simulink model "project_part4_simulink"  (R2025b)
settings: Solver=VariableStepAuto  StartTime=0.0  StopTime=60000  RelTol=1e-3
values from neighbouring files (symbols this model uses):
  denLL = [1 1.14727809e-02 9.96311098e-07]    [Projectpart4_matlab.m]
  Kd = 7.622663874609e-03    (= 0.00762266387461)    [Projectpart4_matlab.m]
  Ki = 2.615765353720e-08    (= 2.61576535372e-08)    [Projectpart4_matlab.m]
  Kp = 5.084451890329e-05    (= 5.08445189033e-05)    [Projectpart4_matlab.m]
  N = 4.500000000000e-02    (= 0.045)    [Projectpart4_matlab.m]
  numLL = [1.73797606e-04 5.57358725e-07 2.53973523e-10]    [Projectpart4_matlab.m]
  Td = 11.7    [Projectpart4_matlab.m]
libraries: slpidlib x10, simulink x2
settings Model: PacingRate=1000  Creator=DELL  LastModifiedBy=renef

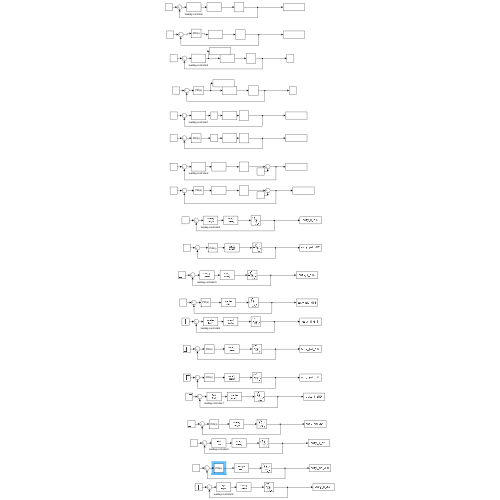
[thumbnail: Simulink's stored preview of the top-level diagram]
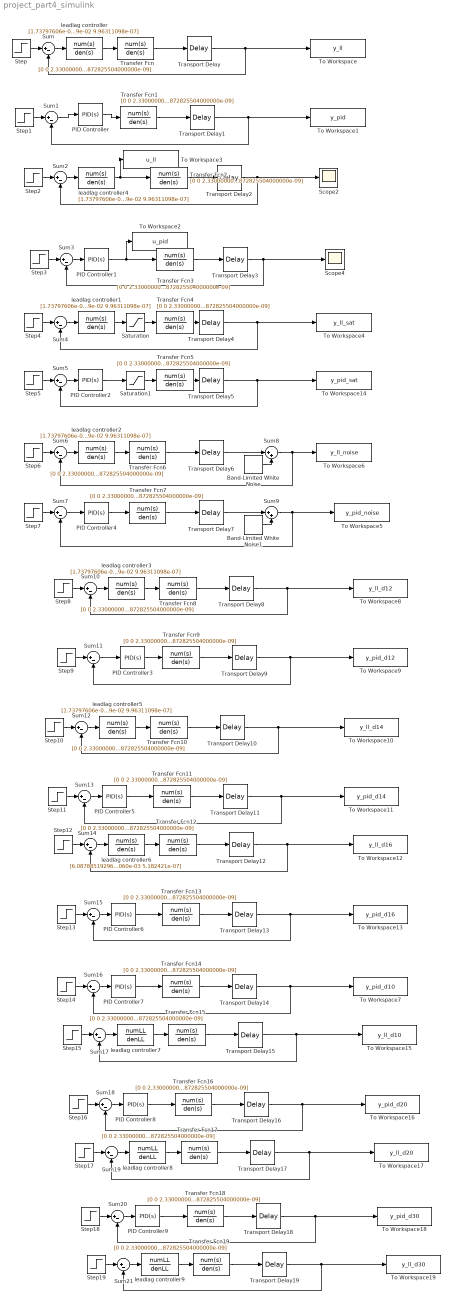
== system project_part4_simulink ==
  Band-Limited White Noise : simulink/Sources/Band-Limited White Noise  Cov=[0.001]  Ts=1  seed=[23341]
  Band-Limited White Noise1 : simulink/Sources/Band-Limited White Noise  Cov=[0.001]  Ts=1  seed=[23341]
  PID Controller{,1..6} (7 alike) : slpidlib/PID Controller  Controller=PID  Form=Parallel  TimeDomain=Continuous-time  UseExternalTs=off  SampleTime=-1  IntegratorMethod=Forward Euler  FilterMethod=Forward Euler  ControllerParametersSource=internal  P=5.084451890329e-05  I=2.615765353720e-08  UseKiTs=off  D=7.622663874609e-03  UseExternalDerivativeSource=off  N=4.500000000000e-02  UseFilter=on  TunerSelectOption=Transfer Function Based (PID Tuner App)  InitialConditionSource=internal  InitialConditionForIntegrator=0  InitialConditionForFilter=0  DifferentiatorICPrevScaledInput=0  ExternalReset=none  TrackingMode=off  Kt=1  LimitOutput=off  SatLimitsSource=internal  UpperSaturationLimit=inf  LowerSaturationLimit=-inf  LinearizeAsGain=on  AntiWindupMode=none  Kb=1  LimitIntegrator=off  UpperIntegratorSaturationLimit=inf  LowerIntegratorSaturationLimit=-inf  POutMin=[]  POutMax=[]  IOutMin=[]  IOutMax=[]  DOutMin=[]  DOutMax=[]  NOutMin=[]  NOutMax=[]  SumOutMin=[]  SumOutMax=[]  SaturationOutMin=[]  SaturationOutMax=[]  PParamMin=[]  PParamMax=[]  IParamMin=[]  IParamMax=[]  DParamMin=[]  DParamMax=[]  NParamMin=[]  NParamMax=[]  KbParamMin=[]  KbParamMax=[]  KtParamMin=[]  KtParamMax=[]  KbOutMin=[]  KbOutMax=[]  KtOutMin=[]  KtOutMax=[]  IntegratorOutMin=[]  IntegratorOutMax=[]  FilterOutMin=[]  FilterOutMax=[]  SumI1OutMin=[]  SumI1OutMax=[]  SumI2OutMin=[]  SumI2OutMax=[]  SumI3OutMin=[]  SumI3OutMax=[]  SumI4OutMin=[]  SumI4OutMax=[]  SumDOutMin=[]  SumDOutMax=[]  DifferentiatorOutMin=[]  DifferentiatorOutMax=[]  FilterDiffOutCoefMin=[]  FilterDiffOutCoefMax=[]  ReciprocalOutMin=[]  ReciprocalOutMax=[]  SumDenOutMin=[]  SumDenOutMax=[]  SumNumOutMin=[]  SumNumOutMax=[]  DivideOutMin=[]  DivideOutMax=[]  UdiffTsProdOutMin=[]  UdiffTsProdOutMax=[]  NTsProdOutMin=[]  NTsProdOutMax=[]  UintegralTsProdOutMin=[]  UintegralTsProdOutMax=[]  UngainTsProdOutMin=[]  UngainTsProdOutMax=[]  ClampingZeroOutDataTypeStr=Inherit: Inherit via back propagation  ClampingZeroOutMin=[]  ClampingZeroOutMax=[]  FilterDenConstantOutDataTypeStr=Inherit: Inherit via back propagation  FilterDenConstantOutMin=[]  FilterDenConstantOutMax=[]  PCopyOutDataTypeStr=Inherit: Inherit via back propagation  PCopyOutMin=[]  PCopyOutMax=[]  NCopyOutDataTypeStr=Inherit: Inherit via back propagation  NCopyOutMin=[]  NCopyOutMax=[]  IntegratorContinuousStateAttributes=''  IntegratorStateMustResolveToSignalObject=off  IntegratorRTWStateStorageClass=Auto  FilterContinuousStateAttributes=''  FilterStateMustResolveToSignalObject=off  FilterRTWStateStorageClass=Auto  ParallelPVariant=InternalParameters  IdealPVariant=Disabled  IVariant=InternalParameters  DVariant=InternalParameters  IntegratorVariant=Continuous  SatVariant=Disabled  AWVariant=Passthrough  PCopyVariant=Disabled  TRVariant=Disabled  FdbkBlocksVariant=Forward  IdealPFdbkVariant=Disabled  SatFdbkVariant=Disabled  DerivativeFilterVariant=ContFilter  NVariant=InternalParameters  NCopyVariant=Disabled  FilterICVariant=InternalICsFilter  IntegratorICVariant=InternalICs  ExternalResetVariant=Disabled  TRSumVariant=Passthrough  SumFdbkVariant=Disabled  SumVariant=Sum_PID  TsampFilterVariant=InternalTs  TsampNgainVariant=Passthrough  TsampIntegralVariant=Disabled_SignalSpec  ExternalSaturationOutDataTypeStr=Inherit: Same as second input  DerivativeSourceVariant=ErrorSignal  PreIntVariant=InternalPreInt
  PID Controller7 : slpidlib/PID Controller  Controller=PID  Form=Parallel  TimeDomain=Continuous-time  UseExternalTs=off  SampleTime=-1  IntegratorMethod=Forward Euler  FilterMethod=Forward Euler  ControllerParametersSource=internal  P=Kp  I=Ki  UseKiTs=off  D=Kd  UseExternalDerivativeSource=off  N=N  UseFilter=on  TunerSelectOption=Transfer Function Based (PID Tuner App)  InitialConditionSource=internal  InitialConditionForIntegrator=0  InitialConditionForFilter=0  DifferentiatorICPrevScaledInput=0  ExternalReset=none  TrackingMode=off  Kt=1  LimitOutput=off  SatLimitsSource=internal  UpperSaturationLimit=inf  LowerSaturationLimit=-inf  LinearizeAsGain=on  AntiWindupMode=none  Kb=1  LimitIntegrator=off  UpperIntegratorSaturationLimit=inf  LowerIntegratorSaturationLimit=-inf  POutMin=[]  POutMax=[]  IOutMin=[]  IOutMax=[]  DOutMin=[]  DOutMax=[]  NOutMin=[]  NOutMax=[]  SumOutMin=[]  SumOutMax=[]  SaturationOutMin=[]  SaturationOutMax=[]  PParamMin=[]  PParamMax=[]  IParamMin=[]  IParamMax=[]  DParamMin=[]  DParamMax=[]  NParamMin=[]  NParamMax=[]  KbParamMin=[]  KbParamMax=[]  KtParamMin=[]  KtParamMax=[]  KbOutMin=[]  KbOutMax=[]  KtOutMin=[]  KtOutMax=[]  IntegratorOutMin=[]  IntegratorOutMax=[]  FilterOutMin=[]  FilterOutMax=[]  SumI1OutMin=[]  SumI1OutMax=[]  SumI2OutMin=[]  SumI2OutMax=[]  SumI3OutMin=[]  SumI3OutMax=[]  SumI4OutMin=[]  SumI4OutMax=[]  SumDOutMin=[]  SumDOutMax=[]  DifferentiatorOutMin=[]  DifferentiatorOutMax=[]  FilterDiffOutCoefMin=[]  FilterDiffOutCoefMax=[]  ReciprocalOutMin=[]  ReciprocalOutMax=[]  SumDenOutMin=[]  SumDenOutMax=[]  SumNumOutMin=[]  SumNumOutMax=[]  DivideOutMin=[]  DivideOutMax=[]  UdiffTsProdOutMin=[]  UdiffTsProdOutMax=[]  NTsProdOutMin=[]  NTsProdOutMax=[]  UintegralTsProdOutMin=[]  UintegralTsProdOutMax=[]  UngainTsProdOutMin=[]  UngainTsProdOutMax=[]  ClampingZeroOutDataTypeStr=Inherit: Inherit via back propagation  ClampingZeroOutMin=[]  ClampingZeroOutMax=[]  FilterDenConstantOutDataTypeStr=Inherit: Inherit via back propagation  FilterDenConstantOutMin=[]  FilterDenConstantOutMax=[]  PCopyOutDataTypeStr=Inherit: Inherit via back propagation  PCopyOutMin=[]  PCopyOutMax=[]  NCopyOutDataTypeStr=Inherit: Inherit via back propagation  NCopyOutMin=[]  NCopyOutMax=[]  IntegratorContinuousStateAttributes=''  IntegratorStateMustResolveToSignalObject=off  IntegratorRTWStateStorageClass=Auto  FilterContinuousStateAttributes=''  FilterStateMustResolveToSignalObject=off  FilterRTWStateStorageClass=Auto  ParallelPVariant=InternalParameters  IdealPVariant=Disabled  IVariant=InternalParameters  DVariant=InternalParameters  IntegratorVariant=Continuous  SatVariant=Disabled  AWVariant=Passthrough  PCopyVariant=Disabled  TRVariant=Disabled  FdbkBlocksVariant=Forward  IdealPFdbkVariant=Disabled  SatFdbkVariant=Disabled  DerivativeFilterVariant=ContFilter  NVariant=InternalParameters  NCopyVariant=Disabled  FilterICVariant=InternalICsFilter  IntegratorICVariant=InternalICs  ExternalResetVariant=Disabled  TRSumVariant=Passthrough  SumFdbkVariant=Disabled  SumVariant=Sum_PID  TsampFilterVariant=InternalTs  TsampNgainVariant=Passthrough  TsampIntegralVariant=Disabled_SignalSpec  ExternalSaturationOutDataTypeStr=Inherit: Same as second input  DerivativeSourceVariant=ErrorSignal  PreIntVariant=InternalPreInt
  PID Controller8 : slpidlib/PID Controller  Controller=PID  Form=Parallel  TimeDomain=Continuous-time  UseExternalTs=off  SampleTime=-1  IntegratorMethod=Forward Euler  FilterMethod=Forward Euler  ControllerParametersSource=internal  P=Kp  I=Ki  UseKiTs=off  D=Kd  UseExternalDerivativeSource=off  N=N  UseFilter=on  TunerSelectOption=Transfer Function Based (PID Tuner App)  InitialConditionSource=internal  InitialConditionForIntegrator=0  InitialConditionForFilter=0  DifferentiatorICPrevScaledInput=0  ExternalReset=none  TrackingMode=off  Kt=1  LimitOutput=off  SatLimitsSource=internal  UpperSaturationLimit=inf  LowerSaturationLimit=-inf  LinearizeAsGain=on  AntiWindupMode=none  Kb=1  LimitIntegrator=off  UpperIntegratorSaturationLimit=inf  LowerIntegratorSaturationLimit=-inf  POutMin=[]  POutMax=[]  IOutMin=[]  IOutMax=[]  DOutMin=[]  DOutMax=[]  NOutMin=[]  NOutMax=[]  SumOutMin=[]  SumOutMax=[]  SaturationOutMin=[]  SaturationOutMax=[]  PParamMin=[]  PParamMax=[]  IParamMin=[]  IParamMax=[]  DParamMin=[]  DParamMax=[]  NParamMin=[]  NParamMax=[]  KbParamMin=[]  KbParamMax=[]  KtParamMin=[]  KtParamMax=[]  KbOutMin=[]  KbOutMax=[]  KtOutMin=[]  KtOutMax=[]  IntegratorOutMin=[]  IntegratorOutMax=[]  FilterOutMin=[]  FilterOutMax=[]  SumI1OutMin=[]  SumI1OutMax=[]  SumI2OutMin=[]  SumI2OutMax=[]  SumI3OutMin=[]  SumI3OutMax=[]  SumI4OutMin=[]  SumI4OutMax=[]  SumDOutMin=[]  SumDOutMax=[]  DifferentiatorOutMin=[]  DifferentiatorOutMax=[]  FilterDiffOutCoefMin=[]  FilterDiffOutCoefMax=[]  ReciprocalOutMin=[]  ReciprocalOutMax=[]  SumDenOutMin=[]  SumDenOutMax=[]  SumNumOutMin=[]  SumNumOutMax=[]  DivideOutMin=[]  DivideOutMax=[]  UdiffTsProdOutMin=[]  UdiffTsProdOutMax=[]  NTsProdOutMin=[]  NTsProdOutMax=[]  UintegralTsProdOutMin=[]  UintegralTsProdOutMax=[]  UngainTsProdOutMin=[]  UngainTsProdOutMax=[]  ClampingZeroOutDataTypeStr=Inherit: Inherit via back propagation  ClampingZeroOutMin=[]  ClampingZeroOutMax=[]  FilterDenConstantOutDataTypeStr=Inherit: Inherit via back propagation  FilterDenConstantOutMin=[]  FilterDenConstantOutMax=[]  PCopyOutDataTypeStr=Inherit: Inherit via back propagation  PCopyOutMin=[]  PCopyOutMax=[]  NCopyOutDataTypeStr=Inherit: Inherit via back propagation  NCopyOutMin=[]  NCopyOutMax=[]  IntegratorContinuousStateAttributes=''  IntegratorStateMustResolveToSignalObject=off  IntegratorRTWStateStorageClass=Auto  FilterContinuousStateAttributes=''  FilterStateMustResolveToSignalObject=off  FilterRTWStateStorageClass=Auto  ParallelPVariant=InternalParameters  IdealPVariant=Disabled  IVariant=InternalParameters  DVariant=InternalParameters  IntegratorVariant=Continuous  SatVariant=Disabled  AWVariant=Passthrough  PCopyVariant=Disabled  TRVariant=Disabled  FdbkBlocksVariant=Forward  IdealPFdbkVariant=Disabled  SatFdbkVariant=Disabled  DerivativeFilterVariant=ContFilter  NVariant=InternalParameters  NCopyVariant=Disabled  FilterICVariant=InternalICsFilter  IntegratorICVariant=InternalICs  ExternalResetVariant=Disabled  TRSumVariant=Passthrough  SumFdbkVariant=Disabled  SumVariant=Sum_PID  TsampFilterVariant=InternalTs  TsampNgainVariant=Passthrough  TsampIntegralVariant=Disabled_SignalSpec  ExternalSaturationOutDataTypeStr=Inherit: Same as second input  DerivativeSourceVariant=ErrorSignal  PreIntVariant=InternalPreInt
  PID Controller9 : slpidlib/PID Controller  Controller=PID  Form=Parallel  TimeDomain=Continuous-time  UseExternalTs=off  SampleTime=-1  IntegratorMethod=Forward Euler  FilterMethod=Forward Euler  ControllerParametersSource=internal  P=Kp  I=Ki  UseKiTs=off  D=Kd  UseExternalDerivativeSource=off  N=N  UseFilter=on  TunerSelectOption=Transfer Function Based (PID Tuner App)  InitialConditionSource=internal  InitialConditionForIntegrator=0  InitialConditionForFilter=0  DifferentiatorICPrevScaledInput=0  ExternalReset=none  TrackingMode=off  Kt=1  LimitOutput=off  SatLimitsSource=internal  UpperSaturationLimit=inf  LowerSaturationLimit=-inf  LinearizeAsGain=on  AntiWindupMode=none  Kb=1  LimitIntegrator=off  UpperIntegratorSaturationLimit=inf  LowerIntegratorSaturationLimit=-inf  POutMin=[]  POutMax=[]  IOutMin=[]  IOutMax=[]  DOutMin=[]  DOutMax=[]  NOutMin=[]  NOutMax=[]  SumOutMin=[]  SumOutMax=[]  SaturationOutMin=[]  SaturationOutMax=[]  PParamMin=[]  PParamMax=[]  IParamMin=[]  IParamMax=[]  DParamMin=[]  DParamMax=[]  NParamMin=[]  NParamMax=[]  KbParamMin=[]  KbParamMax=[]  KtParamMin=[]  KtParamMax=[]  KbOutMin=[]  KbOutMax=[]  KtOutMin=[]  KtOutMax=[]  IntegratorOutMin=[]  IntegratorOutMax=[]  FilterOutMin=[]  FilterOutMax=[]  SumI1OutMin=[]  SumI1OutMax=[]  SumI2OutMin=[]  SumI2OutMax=[]  SumI3OutMin=[]  SumI3OutMax=[]  SumI4OutMin=[]  SumI4OutMax=[]  SumDOutMin=[]  SumDOutMax=[]  DifferentiatorOutMin=[]  DifferentiatorOutMax=[]  FilterDiffOutCoefMin=[]  FilterDiffOutCoefMax=[]  ReciprocalOutMin=[]  ReciprocalOutMax=[]  SumDenOutMin=[]  SumDenOutMax=[]  SumNumOutMin=[]  SumNumOutMax=[]  DivideOutMin=[]  DivideOutMax=[]  UdiffTsProdOutMin=[]  UdiffTsProdOutMax=[]  NTsProdOutMin=[]  NTsProdOutMax=[]  UintegralTsProdOutMin=[]  UintegralTsProdOutMax=[]  UngainTsProdOutMin=[]  UngainTsProdOutMax=[]  ClampingZeroOutDataTypeStr=Inherit: Inherit via back propagation  ClampingZeroOutMin=[]  ClampingZeroOutMax=[]  FilterDenConstantOutDataTypeStr=Inherit: Inherit via back propagation  FilterDenConstantOutMin=[]  FilterDenConstantOutMax=[]  PCopyOutDataTypeStr=Inherit: Inherit via back propagation  PCopyOutMin=[]  PCopyOutMax=[]  NCopyOutDataTypeStr=Inherit: Inherit via back propagation  NCopyOutMin=[]  NCopyOutMax=[]  IntegratorContinuousStateAttributes=''  IntegratorStateMustResolveToSignalObject=off  IntegratorRTWStateStorageClass=Auto  FilterContinuousStateAttributes=''  FilterStateMustResolveToSignalObject=off  FilterRTWStateStorageClass=Auto  ParallelPVariant=InternalParameters  IdealPVariant=Disabled  IVariant=InternalParameters  DVariant=InternalParameters  IntegratorVariant=Continuous  SatVariant=Disabled  AWVariant=Passthrough  PCopyVariant=Disabled  TRVariant=Disabled  FdbkBlocksVariant=Forward  IdealPFdbkVariant=Disabled  SatFdbkVariant=Disabled  DerivativeFilterVariant=ContFilter  NVariant=InternalParameters  NCopyVariant=Disabled  FilterICVariant=InternalICsFilter  IntegratorICVariant=InternalICs  ExternalResetVariant=Disabled  TRSumVariant=Passthrough  SumFdbkVariant=Disabled  SumVariant=Sum_PID  TsampFilterVariant=InternalTs  TsampNgainVariant=Passthrough  TsampIntegralVariant=Disabled_SignalSpec  ExternalSaturationOutDataTypeStr=Inherit: Same as second input  DerivativeSourceVariant=ErrorSignal  PreIntVariant=InternalPreInt
  Saturation : Saturate  UpperLimit=2e-5  LowerLimit=0
  Saturation1 : Saturate  UpperLimit=2e-5  LowerLimit=0
  Scope2 : Scope
      settings: ActiveDisplayYMinimum=-1  ActiveDisplayYMaximum=1  DataLoggingVariableName=ScopeData2
  Scope4 : Scope
      settings: ActiveDisplayYMinimum=-1  ActiveDisplayYMaximum=1  DataLoggingVariableName=ScopeData4
  Step{,1..19} (20 alike) : Step  Time=0  SampleTime=0
  Sum{,1..7,10..21} (20 alike) : Sum  Inputs=|+-
  Sum8 : Sum  Inputs=|++
  Sum9 : Sum  Inputs=|++
  To Workspace : ToWorkspace  VariableName=y_ll  SaveFormat=Structure With Time  SampleTime=-1
  To Workspace1 : ToWorkspace  VariableName=y_pid  SaveFormat=Structure With Time  SampleTime=-1
  To Workspace10 : ToWorkspace  VariableName=y_ll_d14  SaveFormat=Structure With Time  SampleTime=-1
  To Workspace11 : ToWorkspace  VariableName=y_pid_d14  SaveFormat=Structure With Time  SampleTime=-1
  To Workspace12 : ToWorkspace  VariableName=y_ll_d16  SaveFormat=Structure With Time  SampleTime=-1
  To Workspace13 : ToWorkspace  VariableName=y_pid_d16  SaveFormat=Structure With Time  SampleTime=-1
  To Workspace14 : ToWorkspace  VariableName=y_pid_sat  SaveFormat=Structure With Time  SampleTime=-1
  To Workspace15 : ToWorkspace  VariableName=y_ll_d10  SaveFormat=Structure With Time  SampleTime=-1
  To Workspace16 : ToWorkspace  VariableName=y_pid_d20  SaveFormat=Structure With Time  SampleTime=-1
  To Workspace17 : ToWorkspace  VariableName=y_ll_d20  SaveFormat=Structure With Time  SampleTime=-1
  To Workspace18 : ToWorkspace  VariableName=y_pid_d30  SaveFormat=Structure With Time  SampleTime=-1
  To Workspace19 : ToWorkspace  VariableName=y_ll_d30  SaveFormat=Structure With Time  SampleTime=-1
  To Workspace2 : ToWorkspace  VariableName=u_pid  SaveFormat=Structure With Time  SampleTime=-1
  To Workspace3 : ToWorkspace  VariableName=u_ll  SaveFormat=Structure With Time  SampleTime=-1
  To Workspace4 : ToWorkspace  VariableName=y_ll_sat  SaveFormat=Structure With Time  SampleTime=-1
  To Workspace5 : ToWorkspace  VariableName=y_pid_noise  SaveFormat=Structure With Time  SampleTime=-1
  To Workspace6 : ToWorkspace  VariableName=y_ll_noise  SaveFormat=Structure With Time  SampleTime=-1
  To Workspace7 : ToWorkspace  VariableName=y_pid_d10  SaveFormat=Structure With Time  SampleTime=-1
  To Workspace8 : ToWorkspace  VariableName=y_ll_d12  SaveFormat=Structure With Time  SampleTime=-1
  To Workspace9 : ToWorkspace  VariableName=y_pid_d12  SaveFormat=Structure With Time  SampleTime=-1
  Transfer Fcn{,1..19} (20 alike) : TransferFcn  Numerator=[0 0 2.330000000000000e-01 3.418110000000001e-02 1.219195800000000e-03]  Denominator=[1.000000000000000e+00 1.287600000000000e-01 3.206690800000000e-03 1.292669832000000e-05 5.872825504000000e-09]
  Transport Delay{,1..7} (8 alike) : TransportDelay  DelayTime=11.7
  Transport Delay10 : TransportDelay  DelayTime=1.4*11.7
  Transport Delay11 : TransportDelay  DelayTime=1.4*11.7
  Transport Delay12 : TransportDelay  DelayTime=1.6*11.7
  Transport Delay13 : TransportDelay  DelayTime=1.6*11.7
  Transport Delay14 : TransportDelay  DelayTime=10*Td
  Transport Delay15 : TransportDelay  DelayTime=10*Td
  Transport Delay16 : TransportDelay  DelayTime=20*Td
  Transport Delay17 : TransportDelay  DelayTime=20*Td
  Transport Delay18 : TransportDelay  DelayTime=30*Td
  Transport Delay19 : TransportDelay  DelayTime=30*Td
  Transport Delay8 : TransportDelay  DelayTime=1.2*11.7
  Transport Delay9 : TransportDelay  DelayTime=1.2*11.7
  leadlag controller{,1..5} (6 alike) : TransferFcn  Numerator=[1.73797606e-04 5.57358725e-07 2.53973523e-10]  Denominator=[1 1.14727809e-02 9.96311098e-07]
  leadlag controller6 : TransferFcn  Numerator=[6.087885192961e-05 2.946536e-07 1.321071e-10]  Denominator=[1 9.142060e-03 5.182421e-07]
  leadlag controller7 : TransferFcn  Numerator=numLL  Denominator=denLL
  leadlag controller8 : TransferFcn  Numerator=numLL  Denominator=denLL
  leadlag controller9 : TransferFcn  Numerator=numLL  Denominator=denLL
  wires:
  PID Controller4/1 -> Transfer Fcn7/1
  Sum/1 -> leadlag controller/1
  Sum8/1 -> To Workspace6/1, Sum6/2
  Band-Limited White Noise/1 -> Sum8/2
  Sum5/1 -> PID Controller2/1
  leadlag controller2/1 -> Transfer Fcn6/1
  Sum1/1 -> PID Controller/1
  Step4/1 -> Sum4/1
  leadlag controller4/1 -> To Workspace3/1, Transfer Fcn2/1
  leadlag controller/1 -> Transfer Fcn/1
  Transport Delay/1 -> To Workspace/1, Sum/2
  Transport Delay2/1 -> Sum2/2, Scope2/1
  Step5/1 -> Sum5/1
  Transport Delay7/1 -> Sum9/1
  Band-Limited White Noise1/1 -> Sum9/2
  PID Controller/1 -> Transfer Fcn1/1
  Transfer Fcn/1 -> Transport Delay/1
  Transfer Fcn7/1 -> Transport Delay7/1
  Step2/1 -> Sum2/1
  Step3/1 -> Sum3/1
  Step6/1 -> Sum6/1
  Transport Delay1/1 -> To Workspace1/1, Sum1/2
  Transfer Fcn2/1 -> Transport Delay2/1
  Transport Delay4/1 -> Sum4/2, To Workspace4/1
  Transfer Fcn5/1 -> Transport Delay5/1
  Saturation1/1 -> Transfer Fcn5/1
  Sum4/1 -> leadlag controller1/1
  Sum2/1 -> leadlag controller4/1
  Transport Delay3/1 -> Sum3/2, Scope4/1
  Transfer Fcn6/1 -> Transport Delay6/1
  PID Controller1/1 -> To Workspace2/1, Transfer Fcn3/1
  Sum3/1 -> PID Controller1/1
  Step/1 -> Sum/1
  Transport Delay5/1 -> To Workspace14/1, Sum5/2
  Step1/1 -> Sum1/1
  Step7/1 -> Sum7/1
  leadlag controller1/1 -> Saturation/1
  PID Controller2/1 -> Saturation1/1
  Transfer Fcn1/1 -> Transport Delay1/1
  Sum9/1 -> Sum7/2, To Workspace5/1
  Sum6/1 -> leadlag controller2/1
  Transfer Fcn4/1 -> Transport Delay4/1
  Transfer Fcn3/1 -> Transport Delay3/1
  Saturation/1 -> Transfer Fcn4/1
  Transport Delay6/1 -> Sum8/1
  Step8/1 -> Sum10/1
  Step9/1 -> Sum11/1
  Transfer Fcn9/1 -> Transport Delay9/1
  Transport Delay9/1 -> To Workspace9/1, Sum11/2
  Transfer Fcn8/1 -> Transport Delay8/1
  Transport Delay8/1 -> To Workspace8/1, Sum10/2
  Sum10/1 -> leadlag controller3/1
  leadlag controller3/1 -> Transfer Fcn8/1
  leadlag controller5/1 -> Transfer Fcn10/1
  Step11/1 -> Sum13/1
  Transport Delay10/1 -> To Workspace10/1, Sum12/2
  Transfer Fcn10/1 -> Transport Delay10/1
  Transport Delay11/1 -> To Workspace11/1, Sum13/2
  Transfer Fcn11/1 -> Transport Delay11/1
  Sum12/1 -> leadlag controller5/1
  Step10/1 -> Sum12/1
  Transfer Fcn12/1 -> Transport Delay12/1
  leadlag controller6/1 -> Transfer Fcn12/1
  Transfer Fcn13/1 -> Transport Delay13/1
  Step12/1 -> Sum14/1
  Transport Delay13/1 -> To Workspace13/1, Sum15/2
  Step13/1 -> Sum15/1
  Transport Delay12/1 -> To Workspace12/1, Sum14/2
  Sum14/1 -> leadlag controller6/1
  Sum7/1 -> PID Controller4/1
  Sum11/1 -> PID Controller3/1
  PID Controller3/1 -> Transfer Fcn9/1
  Sum13/1 -> PID Controller5/1
  PID Controller5/1 -> Transfer Fcn11/1
  PID Controller6/1 -> Transfer Fcn13/1
  Sum15/1 -> PID Controller6/1
  Transfer Fcn15/1 -> Transport Delay15/1
  leadlag controller7/1 -> Transfer Fcn15/1
  Sum16/1 -> PID Controller7/1
  Sum17/1 -> leadlag controller7/1
  Transport Delay15/1 -> To Workspace15/1, Sum17/2
  PID Controller7/1 -> Transfer Fcn14/1
  Transport Delay14/1 -> To Workspace7/1, Sum16/2
  Step15/1 -> Sum17/1
  Transfer Fcn14/1 -> Transport Delay14/1
  Step14/1 -> Sum16/1
  Transfer Fcn17/1 -> Transport Delay17/1
  leadlag controller8/1 -> Transfer Fcn17/1
  Sum18/1 -> PID Controller8/1
  Sum19/1 -> leadlag controller8/1
  Transport Delay17/1 -> To Workspace17/1, Sum19/2
  PID Controller8/1 -> Transfer Fcn16/1
  Transport Delay16/1 -> To Workspace16/1, Sum18/2
  Step17/1 -> Sum19/1
  Transfer Fcn16/1 -> Transport Delay16/1
  Step16/1 -> Sum18/1
  Transfer Fcn19/1 -> Transport Delay19/1
  leadlag controller9/1 -> Transfer Fcn19/1
  Sum20/1 -> PID Controller9/1
  Sum21/1 -> leadlag controller9/1
  Transport Delay19/1 -> To Workspace19/1, Sum21/2
  PID Controller9/1 -> Transfer Fcn18/1
  Transport Delay18/1 -> To Workspace18/1, Sum20/2
  Step19/1 -> Sum21/1
  Transfer Fcn18/1 -> Transport Delay18/1
  Step18/1 -> Sum20/1
